simulink model "main"  (R2018b)
settings: Solver=FixedStepDiscrete  StartTime=0.0  StopTime=inf  RelTol=1e-3
values from neighbouring files (symbols this model uses):
  N = n_vector(n)    [perf.m]    (also in var.m = 64)
  pilote = N*taux_pilote    [perf.m]    (also in var.m = 16)
  prefix = 3    [perf.m]    (also in var.m)
  taux_pilote = taux_pilote_vector(taux)    [perf.m]    (also in var.m = 0.25)
  Ts = 3.2e-6    (= 3.2e-06)    [perf.m]    (also in var.m)
undefined symbols (not defined in the file or in its folder): doppler, j, palier
libraries: dspindex x4, commchan3 x2, dspxfrm3 x2, commdigbbndpm3 x2, commsdrhw_v2 x2, commsink2 x1, commrandsrc3 x1
settings Model: SimulationMode=accelerator  Creator=speychet  LastModifiedBy=titou
settings SolverCC: AutoInsertRateTranBlk=on
settings DataIOCC: LimitDataPoints=on  SaveOutput=off  SignalLogging=off  SaveTime=off
settings OptimizationCC: EfficientMapNaN2IntZero=off  LifeSpan=inf
settings DebuggingCC: AlgebraicLoopMsg=error  SingleTaskRateTransMsg=error  AllowSymbolicDim=off  SFUnexpectedBacktrackingDiag=warning  SFNoUnconditionalDefaultTransitionDiag=warning  SFExecutionAtInitializationDiag=none
settings HardwareCC: TargetBitPerPointer=64  TargetBitPerSizeT=64  TargetBitPerPtrDiffT=64  TargetLongLongMode=on  TargetIntDivRoundTo=Zero  TargetEndianess=LittleEndian  TargetWordSize=64  TargetHWDeviceType=MATLAB Host  ProdEqTarget=off
settings SFSimCC: SimUseLocalCustomCode=off
settings CodeAppCC: MaxIdLength=128
settings GRTTargetCC: TargetLangStandard=C89/C90 (ANSI)  CombineOutputUpdateFcns=off  GRTInterface=on

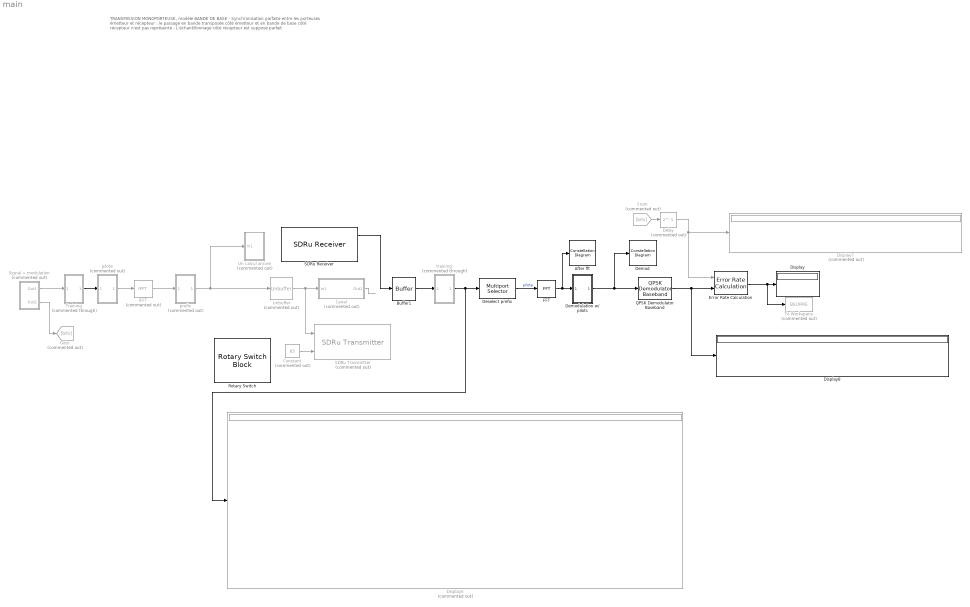
== system main ==
  note: TRANSMISSION MONOPORTEUSE, modèle BANDE DE BASE
      |
      | - Synchronisation parfaite entre les porteuses émetteur et récepteur : le passage en bande transposée côté émetteur et en bande de base côté récepteur n'est pas représenté
      |
      | - L'échantillonnage côté récepteur est supposé parfait
  After fft : ConstellationDiagram
  Buffer1 : Buffer  N=N+pilote+prefix  OutputFrames=off
  Canal : Subsystem  Commented=on
  Constant : Constant  Commented=on  Value=65
  Delay : Delay  Commented=on  DelayLength=1
  Demod : ConstellationDiagram
  Demodulation w/ pilots : Subsystem
  Deselect prefix : dspindex/Multiport Selector  rowsOrCols=Rows  idxCellArray={ (prefix+1) : (N+pilote+prefix) }  idxErrMode=Clip Index
  Display : Display
  Display5 : Display  Commented=on
  Display7 : Display  Commented=on
  Display8 : Display
  Error Rate Calculation : commsink2/Error Rate Calculation  N=0  st_delay=0  cp_mode=Entire frame  subframe=[]  PMode=Port  WsName=ErrorVec  RsMode2=off  stop=off  numErr=100  maxBits=1e6
      settings: SourceProductName=Communications Toolbox
  FFT : dspxfrm3/FFT  FFTImplementation=Auto  CompMethod=Table lookup  TableOpt=NEW  TableOptActive=Speed  BitRevOrder=off  Normalize=off  InheritFFTLength=on  FFTLength=64  WrapInput=on  roundingMode=Floor  overflowMode=off  firstCoeffDataTypeStr=Inherit: Same word length as input  firstCoeffLastDataTypeStr=Inherit: Same word length as input  outputMin=[]  outputMax=[]
  From : From  Commented=on  GotoTag=bits
  Goto : Goto  Commented=on  GotoTag=bits
  IFFT : dspxfrm3/IFFT  Commented=on  FFTImplementation=Auto  CompMethod=Table lookup  TableOpt=NEW  TableOptActive=Speed  BitRevOrder=off  cs_in=off  Normalize=on  InheritFFTLength=on  FFTLength=64  WrapInput=on  mode=Complex  outSamplingMode=Sample based  roundingMode=Floor  overflowMode=off  firstCoeffDataTypeStr=Inherit: Same word length as input  firstCoeffLastDataTypeStr=Inherit: Same word length as input  outputMin=[]  outputMax=[]
      settings: SourceProductName=DSP System Toolbox
  QPSK Demodulator Baseband : commdigbbndpm3/QPSK Demodulator Baseband  OutType=Bit  DecType=Hard decision  VarSource=Dialog  Variance=1  Dec=Gray  Ph=pi/4  outDtype1=Inherit via internal rule  outDtype2=Inherit via internal rule  derotateFactorWordLen=16  derotateFactorDataTypeStr=Inherit: Same word length as input  derotateFactorLastDataTypeStr=Inherit: Same word length as input
      settings: SourceProductName=Communications Toolbox
  Rotary Switch : RotarySwitchBlock  WebBlockId=200
      settings: Values={{'69', '65', '70', '75', '80'}, [60 65 70 75 80]}
  SDRu Receiver : commsdrhw_v2/SDRu Receiver  rxtx=rx  initializeIPAddress=0  devMap=0  USRP2_IP=192.168.10.2  USRP_IP_X300=192.168.10.2  USRP_IP_X310=192.168.10.2  USRP_serialNumB200=No devices found  USRP_serialNumB210=30CEEA9  platform=B210  prevPlatform=B210  lastIPAddressPopup=192.168.10.2  USRP_ID=30CEEA9  LastIPAddress=192.168.10.2  ChannelMapping=1  centerFrequencySrc=Dialog  centerFrequency=5.2e9  loOffsetSrc=Dialog  loOffset=1e6  gainSrc=Dialog  gain=60  PPSSource=Internal  clockSource=Internal  masterClkRateParam=20000000  masterClkRateB200=32e6  masterClkRateB210=20e6  masterClkRateX300=200e6  masterClkRateX310=200e6  masterClkRate=100e6  decimInterpSrc=Dialog  decimInterp=1  USRP2_IP_NUM=[51 48 67 69 69 65 57]  TransportDataType=int16  overrunUnderrunPort=off  sampleTime=1  outputDatatype=double  frameLength=N+prefix+pilote  HOST_DATA_PORT=0  HOST_CONTROL_PORT=0  USRP2_DATA_PORT=0  USRP2_CONTROL_PORT=0  bufferMode=Continuous streaming  EnableBurstMode=on  NumFramesInBurst=100
      settings: SourceProductName=Communications System Toolbox Support Package for USRP(R) Radio  SourceProductBaseCode=USRP
  SDRu Transmitter : commsdrhw_v2/SDRu Transmitter  Commented=on  rxtx=tx  initializeIPAddress=0  devMap=0  USRP2_IP=192.168.10.2  USRP_IP_X300=192.168.10.2  USRP_IP_X310=192.168.10.2  USRP_serialNumB200=No devices found  USRP_serialNumB210=30CEE7A  platform=B210  prevPlatform=B210  lastIPAddressPopup=192.168.10.2  USRP_ID=30CEE7A  LastIPAddress=192.168.10.2  ChannelMapping=1  centerFrequencySrc=Dialog  centerFrequency=5.2e9  loOffsetSrc=Dialog  loOffset=1e6  gainSrc=Input port  gain=60  PPSSource=Internal  clockSource=Internal  masterClkRateParam=5000000  masterClkRateB200=32e6  masterClkRateB210=2e6  masterClkRateX300=120e6  masterClkRateX310=120e6  decimInterpSrc=Dialog  decimInterp=10  USRP2_IP_NUM=[51 48 67 69 69 55 65]  frameLength=362  TransportDataType=int16  outputDatatype=Same as transport data type  overrunUnderrunPort=off  sampleTime=1  dboardInfo=|  HOST_DATA_PORT=30000  HOST_CONTROL_PORT=30001  USRP2_DATA_PORT=32769  USRP2_CONTROL_PORT=32768  bufferMode=Continuous streaming  EnableBurstMode=off  NumFramesInBurst=100
      | dbid: 0
      |           dbName: 'no db found'
      |          freqMin: 0
      |          freqMax: 0
      |          gainMin: 0
      |          gainMax: 0
      |     gainStepSize: 0
      settings: SourceProductName=Communications System Toolbox Support Package for USRP(R) Radio  SourceProductBaseCode=USRP
  Signal + modulation : Subsystem  Commented=on
  To Workspace : ToWorkspace  Commented=on  VariableName=BEURRE  SaveFormat=Timeseries  SampleTime=-1
  Training : Subsystem  Commented=through
  Un calcul ancien : Subsystem  Commented=on
  Unbuffer : Unbuffer  Commented=on
  pilote : Subsystem  Commented=on
  prefix : Subsystem  Commented=on
  training : Subsystem  Commented=through
  wires:
  Error Rate Calculation/1 -> To Workspace/1, Display/1
  From/1 -> Delay/1
  Delay/1 -> Error Rate Calculation/1, Display7/1
  QPSK Demodulator Baseband/1 -> Error Rate Calculation/2, Display8/1
  Deselect prefix/1 -> FFT/1  "pilote"
  Signal + modulation/1(Out1) -> Training/1(In1)
  Training/1(Out1) -> pilote/1(In1)
  pilote/1(Out1) -> IFFT/1
  prefix/1(Out1) -> Un calcul ancien/1(In1), Unbuffer/1
  IFFT/1 -> prefix/1(In1)
  training/1(Out1) -> Display5/1, Deselect prefix/1
  Buffer1/1 -> training/1(In1)
  Demodulation w/ pilots/1(Out1) -> Demod/1, QPSK Demodulator Baseband/1
  FFT/1 -> After fft/1, Demodulation w/ pilots/1(In1)
  Signal + modulation/2(Out2) -> Goto/1
  Unbuffer/1 -> SDRu Transmitter/1, Canal/1(In1)
  Constant/1 -> SDRu Transmitter/2
  SDRu Receiver/1 -> Buffer1/1
  Canal/1(Out1) -> ?

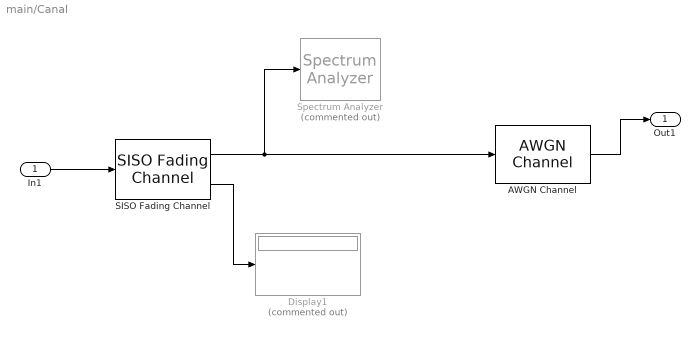
== system main/Canal ==
  In1 : Inport
  AWGN Channel : commchan3/AWGN Channel  InputProcessing=Columns as channels (frame based)  seed=67  noiseMode="Signal to noise ratio  (SNR)"  EbNodB=10  EsNodB=10  SNRdB=SNR  bitsPerSym=1  Ps=0.01397  Tsym=1  variance=1
      settings: SourceProductName=Communications Toolbox
  Display1 : Display  Commented=on
  SISO Fading Channel : commchan3/SISO Fading Channel  InheritSampleRate=on  SampleRate=1  PathDelays=[0 2*Ts/(N+pilote+prefix) 3*Ts/(N+pilote+prefix)]  AveragePathGains=[0 -3 -6]  NormalizePathGains=on  FadingDistribution=Rayleigh  KFactor=3  DirectPathDopplerShift=0  DirectPathInitialPhase=0  MaximumDopplerShift=100  DopplerSpectrum=doppler('Jakes')  ChannelInterpolationMethod=Polyphase  RandomStream=mt19937ar with seed  RandomNumGenerator=mt19937ar  Seed=randi(1000)  PathGainsOutputPort=on  ChannelFilterDelayOutputPort=off  SimulateUsing=Code generation  Visualization=Off  PathsForDopplerDisplay=1  SamplesToDisplay=25%
      settings: SourceProductName=Communications Toolbox
  Spectrum Analyzer : SpectrumAnalyzer  Commented=on
  Out1 : Outport
  wires:
  SISO Fading Channel/2 -> Display1/1
  SISO Fading Channel/1 -> Spectrum Analyzer/1, AWGN Channel/1
  AWGN Channel/1 -> Out1/1
  In1/1 -> SISO Fading Channel/1

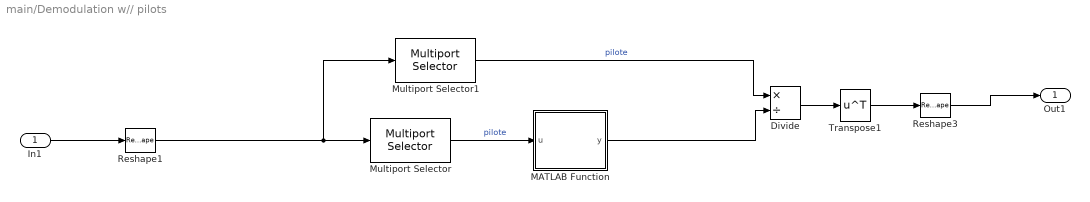
== system main/Demodulation w// pilots ==
  In1 : Inport
  Divide : Product  Inputs=*/
  MATLAB Function : MATLAB Function  TreatAsAtomicUnit=on
  Multiport Selector : dspindex/Multiport Selector  rowsOrCols=Rows  idxCellArray={ pilote+1 }  idxErrMode=Clip Index
  Multiport Selector1 : dspindex/Multiport Selector  rowsOrCols=Rows  idxCellArray={ 1 : (1/taux_pilote) }  idxErrMode=Clip Index
  Reshape1 : Reshape  OutputDimensionality=Customize  OutputDimensions=[ (1/taux_pilote)+1, pilote]
  Reshape3 : Reshape  OutputDimensions=[N,1]
  Transpose1 : Math  Operator=transpose  SaturateOnIntegerOverflow=on
  Out1 : Outport
  wires:
  MATLAB Function/1(y) -> Divide/2
  Reshape1/1 -> Multiport Selector1/1, Multiport Selector/1
  Reshape3/1 -> Out1/1
  Multiport Selector/1 -> MATLAB Function/1(u)  "pilote"
  Divide/1 -> Transpose1/1
  Transpose1/1 -> Reshape3/1
  In1/1 -> Reshape1/1
  Multiport Selector1/1 -> Divide/1  "pilote"

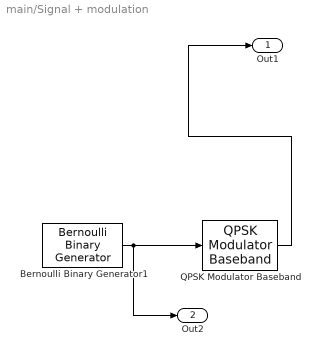
== system main/Signal + modulation ==
  Bernoulli Binary Generator1 : commrandsrc3/Bernoulli Binary Generator  ProbabilityOfZero=0.5  SeedSource=Auto  Seed=0  SampleTime=Ts/(N*2)  SamplesPerFrame=N*2  OutputDataType=double  SimulateUsing=Code generation
      settings: SourceProductName=Communications Toolbox
  QPSK Modulator Baseband : commdigbbndpm3/QPSK Modulator Baseband  InType=Bit  Enc=Gray  Ph=pi/4  outDtype=double  outWordLen=16  outUDDataType=sfix(16)  outFracLenMode=Best precision  outFracLen=15  outDataTypeStr=double  outLastDataTypeStr=double
      settings: SourceProductName=Communications Toolbox
  Out1 : Outport
  Out2 : Outport  Port=2
  wires:
  Bernoulli Binary Generator1/1 -> Out2/1, QPSK Modulator Baseband/1
  QPSK Modulator Baseband/1 -> Out1/1

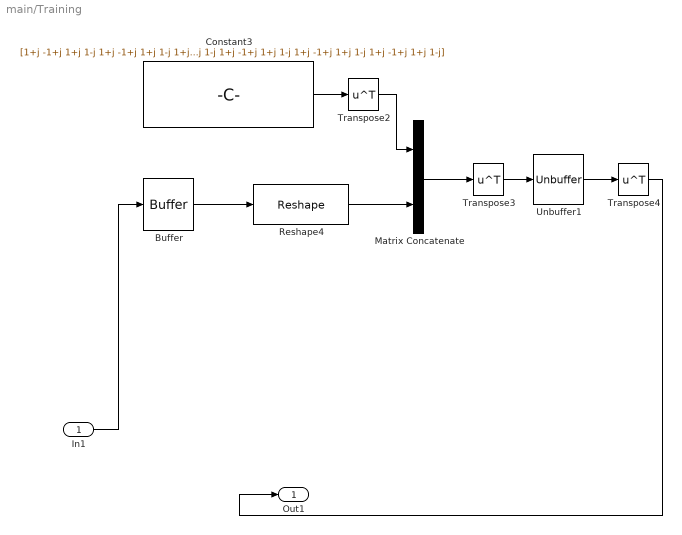
== system main/Training ==
  In1 : Inport
  Buffer : Buffer  N=N*9  OutputFrames=off
  Constant3 : Constant  Value=[1+j -1+j 1+j 1-j 1+j -1+j 1+j 1-j 1+j -1+j 1+j 1-j 1+j -1+j 1+j 1-j 1+j -1+j 1+j 1-j 1+j -1+j 1+j 1-j 1+j -1+j 1+j 1-j 1+j -1+j 1+j 1-j 1+j -1+j 1+j 1-j 1+j -1+j 1+j 1-j 1+j -1+j 1+j 1-j 1+j -1+j 1+j 1-j 1+j -1+j 1+j 1-j 1+j -1+j 1+j 1-j 1+j -1+j 1+j 1-j 1+j -1+j 1+j 1-j]  VectorParams1D=off
  Matrix Concatenate : Concatenate  Mode=Multidimensional array  ConcatenateDimension=2
  Reshape4 : Reshape  OutputDimensionality=Customize  OutputDimensions=[N,9]
  Transpose2 : Math  Operator=transpose  SaturateOnIntegerOverflow=on
  Transpose3 : Math  Operator=transpose  SaturateOnIntegerOverflow=on
  Transpose4 : Math  Operator=transpose  SaturateOnIntegerOverflow=on
  Unbuffer1 : Unbuffer
  Out1 : Outport
  wires:
  Reshape4/1 -> Matrix Concatenate/2
  Unbuffer1/1 -> Transpose4/1
  Transpose2/1 -> Matrix Concatenate/1
  In1/1 -> Buffer/1
  Transpose3/1 -> Unbuffer1/1
  Matrix Concatenate/1 -> Transpose3/1
  Transpose4/1 -> Out1/1
  Buffer/1 -> Reshape4/1
  Constant3/1 -> Transpose2/1

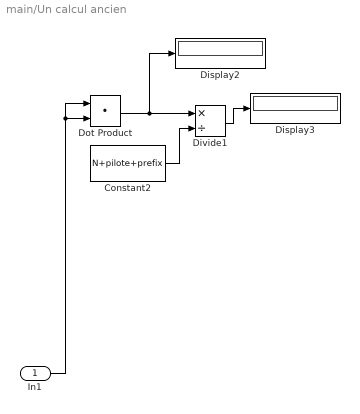
== system main/Un calcul ancien ==
  In1 : Inport
  Constant2 : Constant  Value=N+pilote+prefix
  Display2 : Display
  Display3 : Display
  Divide1 : Product  Inputs=*/
  Dot Product : DotProduct  InputSameDT=on  OutDataTypeStr=Inherit: Inherit via internal rule
  wires:
  Dot Product/1 -> Display2/1, Divide1/1
  Constant2/1 -> Divide1/2
  Divide1/1 -> Display3/1
  In1/1 -> Dot Product/1, Dot Product/2

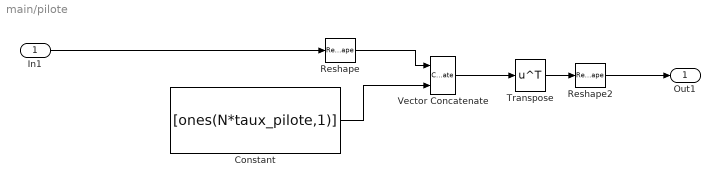
== system main/pilote ==
  In1 : Inport
  Constant : Constant  Value=[ones(N*taux_pilote,1)]  VectorParams1D=off
  Reshape : Reshape  OutputDimensionality=Customize  OutputDimensions=[N*taux_pilote,1/taux_pilote]
  Reshape2 : Reshape  OutputDimensions=[N+(N*taux_pilote),1]
  Transpose : Math  Operator=transpose  SaturateOnIntegerOverflow=on
  Vector Concatenate : Concatenate  Mode=Multidimensional array  ConcatenateDimension=2
  Out1 : Outport
  wires:
  Constant/1 -> Vector Concatenate/2
  Transpose/1 -> Reshape2/1
  In1/1 -> Reshape/1
  Reshape/1 -> Vector Concatenate/1
  Vector Concatenate/1 -> Transpose/1
  Reshape2/1 -> Out1/1

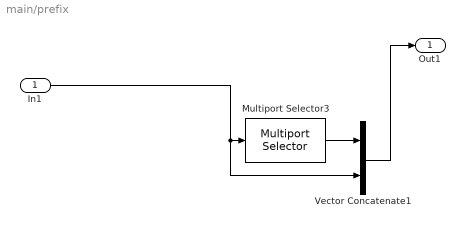
== system main/prefix ==
  In1 : Inport
  Multiport Selector3 : dspindex/Multiport Selector  rowsOrCols=Rows  idxCellArray={ N+pilote-prefix+1 : N+pilote }  idxErrMode=Clip Index
  Vector Concatenate1 : Concatenate  Mode=Multidimensional array
  Out1 : Outport
  wires:
  Vector Concatenate1/1 -> Out1/1
  Multiport Selector3/1 -> Vector Concatenate1/1
  In1/1 -> Multiport Selector3/1, Vector Concatenate1/2

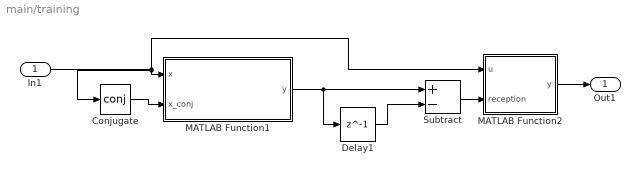
== system main/training ==
  In1 : Inport
  Conjugate : Math  Operator=conj  RndMeth=Zero  SaturateOnIntegerOverflow=on
  Delay1 : Delay  DelayLength=1
  MATLAB Function1 : MATLAB Function  TreatAsAtomicUnit=on
  MATLAB Function2 : MATLAB Function  TreatAsAtomicUnit=on
  Subtract : Sum  Inputs=+-
  Out1 : Outport
  wires:
  Delay1/1 -> Subtract/2
  MATLAB Function1/1(y) -> Delay1/1, Subtract/1
  MATLAB Function2/1(y) -> Out1/1
  Subtract/1 -> MATLAB Function2/2(reception)
  In1/1 -> MATLAB Function2/1(u), Conjugate/1, MATLAB Function1/1(x)
  Conjugate/1 -> MATLAB Function1/2(x_conj)

== matlab function main/training/MATLAB Function1 ==
  data: x input; y output; x_conj input; N parameter
function y = fcn(x, x_conj, N)
s = 0 + 0j;
s1 =-0.0647 - 0.0460j;
for j=1:(N/2)
    s = s + x_conj(j) * x(j+N/2);
end
% if abs(s) >= abs(s1)
%     reception = 1;
%     disp("oui");
% end
    
disp(s);


y = s;

== matlab function main/Demodulation w// pilots/MATLAB Function ==
  data: u input; y output; N parameter; taux_pilote parameter
function y = fcn(u, N, taux_pilote)
tempon = complex(zeros(1/taux_pilote,N*taux_pilote),0);
for row=1:1/taux_pilote
    for column=1:N*taux_pilote - 1
        tempon(row,column+1) = ((u(1,column+1)-u(1,column))*(row/(1/taux_pilote))) + u(1,column);
%         if row == 1
%             tempon(row,column) = u(1,column);
%         end
%         if row == N*taux_pilote
%             tempon(row,column) = u(1,taux_pilotes);
%         end
        if column == 1
            tempon(row,column) = u(1,column);
        end
    end
end
% for row=1:1/taux_pilote
%     tempon(row,N*taux_pilote-1)= u(1,row);
% end
% disp('u =');
% disp(u);
% disp('tempon =');
% disp(tempon);


y = tempon;

== matlab function main/training/MATLAB Function2 ==
  data: u input; y output; reception input; N parameter; pilote parameter; prefix parameter; palier parameter
function y = fcn(u, reception, N, pilote, prefix, palier)
if reception == 0
    palier = 1;
end
if palier == 1
    disp("yes");
    y = u;
else
    y = zeros(N+pilote+prefix,1);
end
